simulink model "ModeloSimulink"  (R2022b)
settings: Solver=VariableStepAuto  StartTime=0.0  StopTime=27.54  RelTol=1e-3
values from neighbouring files (symbols this model uses):
  A = theta(:,1:end-1)    [Estimacion2.m]    (also in measured_data.m)
  B = (theta(:,end))    [Estimacion2.m]    (also in measured_data.m = theta(:,end))
settings Model: Creator=unam-  LastModifiedBy=unam-

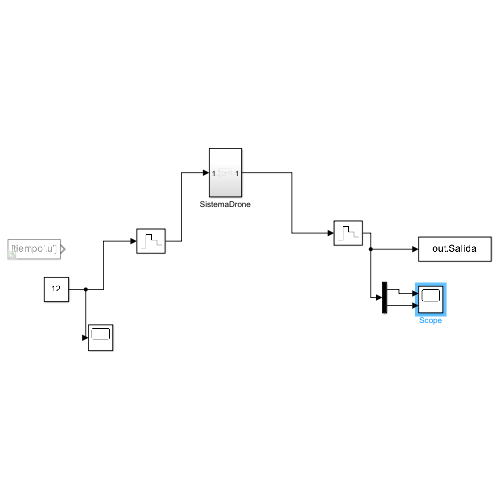
[thumbnail: Simulink's stored preview of the top-level diagram]
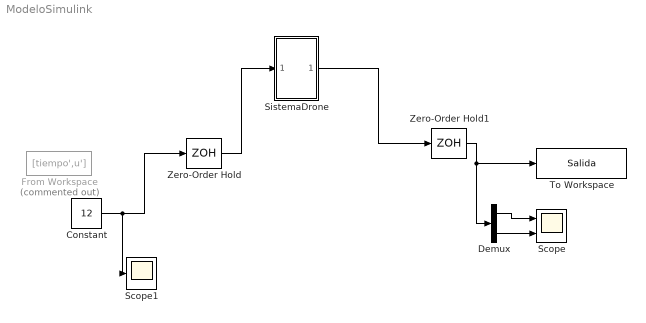
== system ModeloSimulink ==
  Constant : Constant  Value=12
  Demux : Demux  Outputs=2
  From Workspace : FromWorkspace  Commented=on  VariableName=[tiempo',u']  SampleTime=5e-3
  Scope : Scope  NumInputPorts=2
  Scope1 : Scope
  SistemaDrone : Subsystem
  To Workspace : ToWorkspace  VariableName=Salida  SaveFormat=Timeseries  SampleTime=5e-3
  Zero-Order Hold : ZeroOrderHold  SampleTime=5e-3
  Zero-Order Hold1 : ZeroOrderHold  SampleTime=5e-3
  wires:
  Zero-Order Hold/1 -> SistemaDrone/1(In1)
  Zero-Order Hold1/1 -> To Workspace/1, Demux/1
  SistemaDrone/1(Out1) -> Zero-Order Hold1/1
  Demux/1 -> Scope/1
  Demux/2 -> Scope/2
  Constant/1 -> Scope1/1, Zero-Order Hold/1

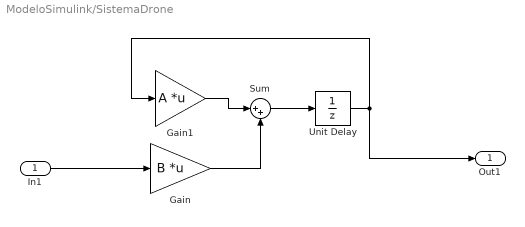
== system ModeloSimulink/SistemaDrone ==
  In1 : Inport
  Gain : Gain  Gain=B  Multiplication=Matrix(K*u)
  Gain1 : Gain  Gain=A  Multiplication=Matrix(K*u)
  Sum : Sum  Inputs=|++
  Unit Delay : UnitDelay  InitialCondition=|  SampleTime=5e-3  HasFrameUpgradeWarning=on
      | [0.00846200000000000;
      | 73.4375000000000]
  Out1 : Outport
  wires:
  Unit Delay/1 -> Out1/1, Gain1/1
  Sum/1 -> Unit Delay/1
  Gain/1 -> Sum/2
  In1/1 -> Gain/1
  Gain1/1 -> Sum/1
